simulink model "Three_Phase_System"  (R2024a)
settings: Solver=VariableStepAuto  StartTime=0.0  StopTime=0.1  RelTol=1e-3
libraries: spsCurrentMeasurementLib x3, spsACVoltageSourceLib x3, spsSeriesRLCBranchLib x3, spsGroundLib x2, spsPowerLib x1, spsVoltageMeasurementLib x1, sps_lib x1
settings Model: Creator=mayan  LastModifiedBy=mayan

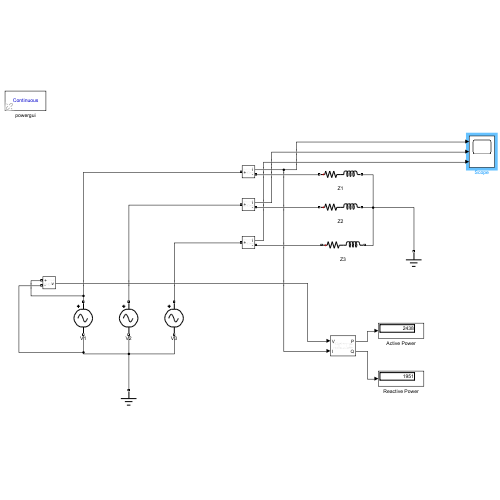
[thumbnail: Simulink's stored preview of the top-level diagram]
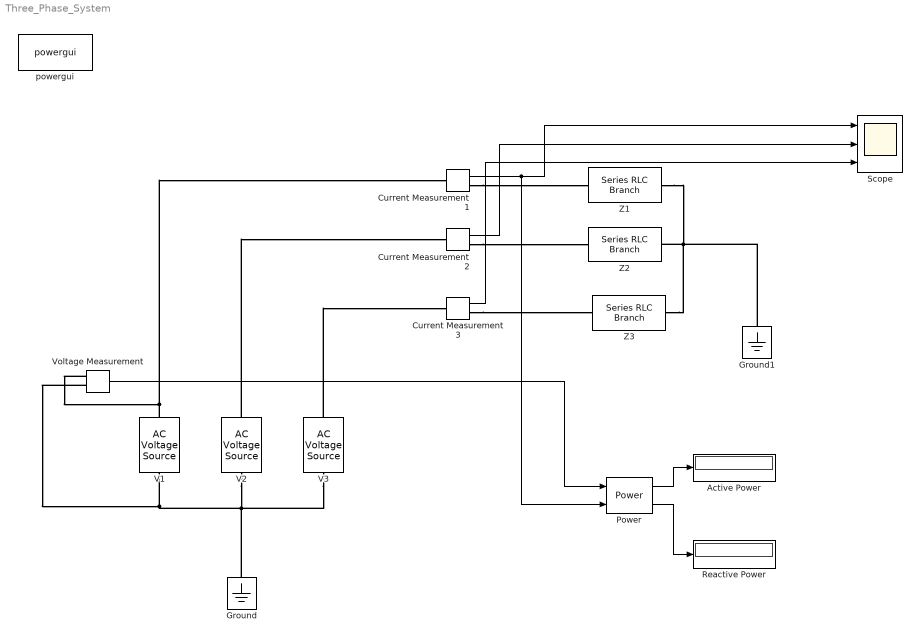
== system Three_Phase_System ==
  Active Power : Display
  Current Measurement1 : spsCurrentMeasurementLib/Current Measurement  PhasorSimulation=off  OutputType=Complex  PSBequivalent=0
  Current Measurement2 : spsCurrentMeasurementLib/Current Measurement  PhasorSimulation=off  OutputType=Complex  PSBequivalent=0
  Current Measurement3 : spsCurrentMeasurementLib/Current Measurement  PhasorSimulation=off  OutputType=Complex  PSBequivalent=0
  Ground : spsGroundLib/Ground  LConnTagsString=a
  Ground1 : spsGroundLib/Ground  LConnTagsString=a
  Power : spsPowerLib/Power  Freq=50  Vinit=[1, 0]  Iinit=[1, 30]  Ts=1e-6
  Reactive Power : Display
  Scope : Scope  NumInputPorts=3
  V1 : spsACVoltageSourceLib/AC Voltage Source  Amplitude=282.8  Phase=0  Frequency=50  SampleTime=1e-6  Measurements=None  BusType=swing  Pref=10e3  Qref=0  Qmin=-inf  Qmax=+inf
  V2 : spsACVoltageSourceLib/AC Voltage Source  Amplitude=282.8  Phase=120  Frequency=50  SampleTime=1e-6  Measurements=None  BusType=swing  Pref=10e3  Qref=0  Qmin=-inf  Qmax=+inf
  V3 : spsACVoltageSourceLib/AC Voltage Source  Amplitude=282.8  Phase=240  Frequency=50  SampleTime=1e-6  Measurements=None  BusType=swing  Pref=10e3  Qref=0  Qmin=-inf  Qmax=+inf
  Voltage Measurement : spsVoltageMeasurementLib/Voltage Measurement  PhasorSimulation=off  OutputType=Complex  PSBequivalent=0
  Z1 : spsSeriesRLCBranchLib/Series RLC Branch  LConnTagsString=__new0  RConnTagsString=__new0  BranchType=RL  Resistance=10  Inductance=0.02546  SetiL0=off  InitialCurrent=0  Capacitance=0  Setx0=off  InitialVoltage=0  Measurements=None
  Z2 : spsSeriesRLCBranchLib/Series RLC Branch  LConnTagsString=__new0  RConnTagsString=__new0  BranchType=RL  Resistance=10  Inductance=0.02546  SetiL0=off  InitialCurrent=0  Capacitance=1e-6  Setx0=off  InitialVoltage=0  Measurements=None
  Z3 : spsSeriesRLCBranchLib/Series RLC Branch  LConnTagsString=__new0  RConnTagsString=__new0  BranchType=RL  Resistance=10  Inductance=0.02546  SetiL0=off  InitialCurrent=0  Capacitance=1e-6  Setx0=off  InitialVoltage=0  Measurements=None
  powergui : sps_lib/powergui  Priority=1  SimulationMode=Continuous  SampleTime=50e-6  frequency=60  Iterations=50  frequencyindice=50  Pbase=100e6  ErrMax=1e-4  UnitsV=kV  UnitsW=MW  buscounter=0  FunctionMessages=off  echomessages=off  EnableUseOfTLC=off  CurrentSourceSwitches=off  DisableSnubberDevices=off  DisableRonSwitches=off  DisableVfSwitches=off  DisplayEquations=off  AutomaticDiscreteSolvers=off  SolverType=Tustin/Backward Euler (TBE)  Interpol=off  ExternalGateDelay=off  methode=off  Ts=100  x0status=blocks  SPID=on  SwTol=0  HookPort=off  NonlinearTolerance=1e-4  nMaxIteration=100  ContinueOnMaxIteration=off  RestoreLinks=warning  ResistiveCurrentMeasurement=off  Frange=[0:2:500]  Ylog=off  Xlog=on  ShowGrid=off  save=off  variable=ZData  structure=0  ZoomFFT=off  StartTime=0.0  cycles=1  DisplayStyle=1  fundamental=60  FreqAxis=off  MaxFrequency=1000  frequencyindicesteady=1  RmsSteady=1  display=off
  wires:
  Power/2 -> Reactive Power/1
  Voltage Measurement/1 -> Power/1
  Current Measurement2/1 -> Scope/2
  Power/1 -> Active Power/1
  Current Measurement1/1 -> Power/2, Scope/1
  Current Measurement3/1 -> Scope/3
  connections:
  V3/LConn1 -- Ground/LConn1 -- V2/LConn1 -- Voltage Measurement/LConn2 -- V1/LConn1
  Z1/RConn1 -- Z2/RConn1 -- Ground1/LConn1 -- Z3/RConn1
  V1/RConn1 -- Voltage Measurement/LConn1 -- Current Measurement1/LConn1
  Current Measurement1/RConn1 -- Z1/LConn1
  V2/RConn1 -- Current Measurement2/LConn1
  Current Measurement2/RConn1 -- Z2/LConn1
  V3/RConn1 -- Current Measurement3/LConn1
  Current Measurement3/RConn1 -- Z3/LConn1
